simulink model "LRMate200Experimentor_ModeController"  (R2015b)
settings: Solver=FixedStepDiscrete  StartTime=0.0  StopTime=10.0  FixedStep=si.itp  RelTol=1e-3
settings Model: Creator=rluser  LastModifiedBy=Chin
settings SolverCC: EnableConcurrentExecution=on
settings DataIOCC: SaveFormat=Array
settings OptimizationCC: BlockReduction=off  OptimizeBlockIOStorage=off  BufferReuse=off  GlobalBufferReuse=off  ExpressionFolding=off  LocalBlockOutputs=off
settings DebuggingCC: SolverPrmCheckMsg=warning
settings HardwareCC: ProdBitPerPointer=32  ProdLargestAtomicFloat=None  ProdWordSize=32  ProdLongLongMode=on  ProdHWDeviceType=Generic->32-bit x86 compatible
settings RTWCC: SystemTargetFile=slrt.tlc  TemplateMakefile=slrt_default_tmf  Description=Simulink Real-Time  RTWCompilerOptimization=on
settings CodeAppCC: MaxIdLength=120
settings SimulinkRealTimeCC: GeneratePreprocessorConditionals=Disable all
settings ConfigComp: CovModelRefEnable=Off  CovSFcnEnable=off

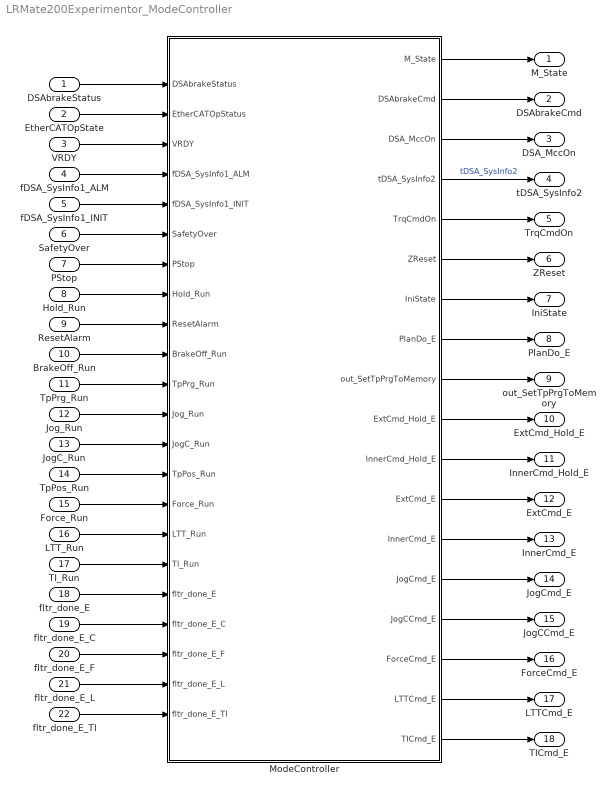
== system LRMate200Experimentor_ModeController ==
  DSAbrakeStatus : Inport
  EtherCATOpState : Inport  Port=2
  VRDY : Inport  Port=3
  fDSA_SysInfo1_ALM : Inport  Port=4
  fDSA_SysInfo1_INIT : Inport  Port=5
  SafetyOver : Inport  Port=6
  PStop : Inport  Port=7
  Hold_Run : Inport  Port=8
  ResetAlarm : Inport  Port=9
  BrakeOff_Run : Inport  Port=10
  TpPrg_Run : Inport  Port=11
  Jog_Run : Inport  Port=12
  JogC_Run : Inport  Port=13
  TpPos_Run : Inport  Port=14
  Force_Run : Inport  Port=15
  LTT_Run : Inport  Port=16
  TI_Run : Inport  Port=17
  fltr_done_E : Inport  Port=18
  fltr_done_E_C : Inport  Port=19
  fltr_done_E_F : Inport  Port=20
  fltr_done_E_L : Inport  Port=21
  fltr_done_E_TI : Inport  Port=22
  ModeController : Stateflow chart  TreatAsAtomicUnit=on
  M_State : Outport
  DSAbrakeCmd : Outport  Port=2
  DSA_MccOn : Outport  Port=3
  tDSA_SysInfo2 : Outport  Port=4
  TrqCmdOn : Outport  Port=5
  ZReset : Outport  Port=6
  IniState : Outport  Port=7
  PlanDo_E : Outport  Port=8
  out_SetTpPrgToMemory : Outport  Port=9
  ExtCmd_Hold_E : Outport  Port=10
  InnerCmd_Hold_E : Outport  Port=11
  ExtCmd_E : Outport  Port=12
  InnerCmd_E : Outport  Port=13
  JogCmd_E : Outport  Port=14
  JogCCmd_E : Outport  Port=15
  ForceCmd_E : Outport  Port=16
  LTTCmd_E : Outport  Port=17
  TICmd_E : Outport  Port=18
  wires:
  ModeController/1(M_State) -> M_State/1
  ModeController/2(DSAbrakeCmd) -> DSAbrakeCmd/1
  ModeController/3(DSA_MccOn) -> DSA_MccOn/1
  ModeController/4(tDSA_SysInfo2) -> tDSA_SysInfo2/1  "tDSA_SysInfo2"
  ModeController/5(TrqCmdOn) -> TrqCmdOn/1
  ModeController/6(ZReset) -> ZReset/1
  DSAbrakeStatus/1 -> ModeController/1(DSAbrakeStatus)
  EtherCATOpState/1 -> ModeController/2(EtherCATOpStatus)
  VRDY/1 -> ModeController/3(VRDY)
  fDSA_SysInfo1_ALM/1 -> ModeController/4(fDSA_SysInfo1_ALM)
  fDSA_SysInfo1_INIT/1 -> ModeController/5(fDSA_SysInfo1_INIT)
  SafetyOver/1 -> ModeController/6(SafetyOver)
  PStop/1 -> ModeController/7(PStop)
  Hold_Run/1 -> ModeController/8(Hold_Run)
  ResetAlarm/1 -> ModeController/9(ResetAlarm)
  BrakeOff_Run/1 -> ModeController/10(BrakeOff_Run)
  TpPrg_Run/1 -> ModeController/11(TpPrg_Run)
  Jog_Run/1 -> ModeController/12(Jog_Run)
  JogC_Run/1 -> ModeController/13(JogC_Run)
  TpPos_Run/1 -> ModeController/14(TpPos_Run)
  Force_Run/1 -> ModeController/15(Force_Run)
  LTT_Run/1 -> ModeController/16(LTT_Run)
  ModeController/7(IniState) -> IniState/1
  ModeController/8(PlanDo_E) -> PlanDo_E/1
  ModeController/9(out_SetTpPrgToMemory) -> out_SetTpPrgToMemory/1
  ModeController/10(ExtCmd_Hold_E) -> ExtCmd_Hold_E/1
  ModeController/11(InnerCmd_Hold_E) -> InnerCmd_Hold_E/1
  ModeController/12(ExtCmd_E) -> ExtCmd_E/1
  ModeController/13(InnerCmd_E) -> InnerCmd_E/1
  ModeController/14(JogCmd_E) -> JogCmd_E/1
  ModeController/15(JogCCmd_E) -> JogCCmd_E/1
  ModeController/16(ForceCmd_E) -> ForceCmd_E/1
  ModeController/17(LTTCmd_E) -> LTTCmd_E/1
  TI_Run/1 -> ModeController/17(TI_Run)
  fltr_done_E/1 -> ModeController/18(fltr_done_E)
  fltr_done_E_C/1 -> ModeController/19(fltr_done_E_C)
  fltr_done_E_F/1 -> ModeController/20(fltr_done_E_F)
  fltr_done_E_L/1 -> ModeController/21(fltr_done_E_L)
  fltr_done_E_TI/1 -> ModeController/22(fltr_done_E_TI)
  ModeController/18(TICmd_E) -> TICmd_E/1

== stateflow chart LRMate200Experimentor_ModeController/ModeController ==
  settings: updateMethod=DISCRETE  sampleTime=si.itp
  state Mode [parallel]
    settings: executionOrder=1
    state WatingForEtherCATReady
      en:M_State=-95;
      TrqCmdOn=0;
      ZReset=1;
      DSAbrakeCmd=0;
      DSA_MccOn=0;
    state INIT_DataCommArea
      en: M_State=-93;
      tDSA_SysInfo2=128;
    state Pstop_State
      state Alarm
        en:M_State=-80;
        TrqCmdOn=0;
        ZReset=1;
      state BrakeOn
        en:M_State=-82;
        DSAbrakeCmd=0;
      state MccOn
        en:M_State=-84;
        DSA_MccOn=1;
      state MccOff
        en:
        M_State=-78;
        DSA_MccOn=0;
      state ResetAlarm1
        en: M_State=-91;
        tDSA_SysInfo2=8;
      state ResetAlarm2
        en: M_State=-89;
        tDSA_SysInfo2=0;
      Alarm -> MccOff
      ResetAlarm2 -> MccOn : [fDSA_SysInfo1_ALM==0]
      ResetAlarm1 -> ResetAlarm2
      Mode.Pstop_State.BrakeOn -> Alarm : after(20,tick)
      (junction 518) -> ResetAlarm1
      MccOff -> (junction 518) : ResetAlarm_E
      MccOn -> (junction 506) : [VRDY==1]
      (junction 506) -> (junction 507)
    state in_stroke
      state Jog_Stopping
        en:JogCmd_E;
        en:M_State=22;
      state BrakeOn
        en:M_State=4;
        DSAbrakeCmd=0;
      state Jogging
        en:JogCmd_E;
        en:M_State=21;
      state JoggingC
        en:JogCCmd_E;
        en:M_State=9921;
      state JogC_Stopping
        en:JogCCmd_E;
        en:M_State=9922;
      state TrqCmdOff
        en:M_State=1;
        TrqCmdOn=0;
        ZReset=1;
      state ForceControl_Stopping
        en:ForceCmd_E;
        en:M_State=9924;
      state ForceControl
        en:ForceCmd_E;
        en:M_State=9923;
      state BrakeOff
        state TrqCmdOn
          en:
          M_State=2;
          TrqCmdOn=1;
          ZReset=0;
        state BrakeOff
          en: DSAbrakeCmd=1;
          M_State=3;
        Mode.in_stroke.BrakeOff.TrqCmdOn -> Mode.in_stroke.BrakeOff.BrakeOff : after(1,tick)
        Mode.in_stroke.BrakeOff.BrakeOff -> (junction 510) : [DSAbrakeStatus==1]
        (junction 510) -> (junction 512) : after(50,tick)
      state LeadThroughTeaching
        en:LTTCmd_E;
        en:M_State=9925;
      state Waiting
        en:M_State=1099;
      state LTT_Stopping
        en:LTTCmd_E;
        en:M_State=9926;
      state TiltInsertion
        en:TICmd_E;
        en:M_State=9927;
      state SetTpPos
        en:  out_SetTpPrgToMemory;
      state TI_Stopping1
        en:TICmd_E;
        en:M_State=9928;
      state IniPosMove_Running1
        en: PlanDo_E;
        InnerCmd_E;
        IniState = 1;
        M_State=9931;
      state SetTpPrg
        en:  out_SetTpPrgToMemory;
      state IniPosMove_Running
        en: PlanDo_E;
        InnerCmd_E;
        IniState = 0;
        M_State=31;
      state Hold_Running
        en:
        M_State=40;
      state TpPrg__Running
        en:
        M_State=33;
        ExtCmd_E;
      Jogging -> Jog_Stopping : Jog_E
      Mode.in_stroke.BrakeOn -> TrqCmdOff : after(10,tick)
      Waiting -> Jogging [order 4] : Jog_E
      Waiting -> JoggingC [order 6] : JogC_E
      Jog_Stopping -> Waiting : [hasChanged(fltr_done_E)]
      Waiting -> Mode.in_stroke.BrakeOn [order 7] : Brake_E
      JoggingC -> JogC_Stopping : JogC_E
      (default) -> (junction 426)
      (junction 426) -> TrqCmdOff
      JogC_Stopping -> Waiting : [hasChanged(fltr_done_E_C)]
      ForceControl -> ForceControl_Stopping : Force_E
      TrqCmdOff -> Mode.in_stroke.BrakeOff.TrqCmdOn : BrakeOff_E
      ForceControl_Stopping -> Waiting : [hasChanged(fltr_done_E_F)]
      Waiting -> ForceControl [order 5] : Force_E
      LeadThroughTeaching -> LTT_Stopping : LTT_E
      Waiting -> LeadThroughTeaching [order 8] : LTT_E
      LTT_Stopping -> Waiting : [hasChanged(fltr_done_E_L)]
      Waiting -> TiltInsertion [order 3] : TI_E
      (junction 188) -> Waiting
      Waiting -> (junction 186) [order 1] : TpPrg_E
      IniPosMove_Running1 -> Waiting : [hasChanged(fltr_done_E)]
      Waiting -> SetTpPos [order 2] : TpPos_E
      TI_Stopping1 -> Waiting : [hasChanged(fltr_done_E_TI)]
      TiltInsertion -> TI_Stopping1 : TI_E
      Hold_Running -> (junction 188) : [hasChanged(fltr_done_E)]
      (junction 177) -> (junction 188)
      (junction 512) -> (junction 180)
      SetTpPos -> IniPosMove_Running1
      (junction 180) -> (junction 177)
      TpPrg__Running -> (junction 177) [order 1] : [hasChanged(fltr_done_E)]
      (junction 598) -> (junction 177)
      (junction 186) -> SetTpPrg
      SetTpPrg -> IniPosMove_Running
      IniPosMove_Running -> Hold_Running [order 2] : Hold_E
          | {InnerCmd_Hold_E;}
      (junction 175) -> Hold_Running
      IniPosMove_Running -> TpPrg__Running [order 1] : [hasChanged(fltr_done_E)]
      TpPrg__Running -> (junction 175) [order 2] : Hold_E
          | {ExtCmd_Hold_E;}
    state out_stroke
      state TrqCmdOff1
        en:M_State=201;
        TrqCmdOn=0;
        ZReset=1;
      state BrakeOn1
        en:M_State=204;
        DSAbrakeCmd=0;
      state BrakeOff1
        state TrqCmdOn
          en:
          M_State=202;
          TrqCmdOn=1;
          ZReset=0;
        state BrakeOff
          en: DSAbrakeCmd=1;
          M_State=203;
        Mode.out_stroke.BrakeOff1.TrqCmdOn -> Mode.out_stroke.BrakeOff1.BrakeOff : after(1,tick)
        Mode.out_stroke.BrakeOff1.BrakeOff -> (junction 524) : [DSAbrakeStatus==1]
        (junction 524) -> (junction 525) : after(50,tick)
      state Waiting1
        en:M_State=210;
      state Jogging1
        en:JogCmd_E;
        en:M_State=221;
      state Jog_Stopping1
        en:JogCmd_E;
        en:M_State=222;
      (default) -> (junction 433)
      (junction 433) -> TrqCmdOff1
      BrakeOn1 -> TrqCmdOff1 : after(10,tick)
      Waiting1 -> BrakeOn1 [order 2] : Brake_E
      TrqCmdOff1 -> Mode.out_stroke.BrakeOff1.TrqCmdOn : BrakeOff_E
      (junction 485) -> (junction 487) [order 1] : [SafetyOver==0]
      Waiting1 -> (junction 485) [order 3] : ResetAlarm_E
      (junction 485) -> Waiting1 [order 2]
      (junction 487) -> (junction 501)
      Waiting1 -> Jogging1 [order 1] : Jog_E
      (junction 461) -> Waiting1
      Jog_Stopping1 -> Waiting1 : [hasChanged(fltr_done_E)]
      Jogging1 -> Jog_Stopping1 : Jog_E
      (junction 525) -> (junction 460)
      (junction 460) -> (junction 461)
      (junction 501) -> (junction 504)
    (default) -> WatingForEtherCATReady
    WatingForEtherCATReady -> INIT_DataCommArea : [EtherCATOpStatus==8]
    INIT_DataCommArea -> (junction 518) : [fDSA_SysInfo1_INIT==1]
    (junction 406) -> Mode.Pstop_State.BrakeOn
    (junction 401) -> (junction 406)
    (junction 507) -> (junction 417)
    (junction 417) -> (junction 423) [order 2]
    (junction 417) -> (junction 419) [order 1] : [SafetyOver==0]
    (junction 423) -> out_stroke : % [SafetyOver==1]
    (junction 419) -> in_stroke
    in_stroke -> (junction 401) [order 1] : PStop_E
    out_stroke -> (junction 401) [order 1] : PStop_E
    (junction 403) -> (junction 401)
    in_stroke -> (junction 403) [order 2] : [fDSA_SysInfo1_ALM==1]
    (junction 439) -> (junction 403)
    in_stroke -> (junction 439) [order 3] : [SafetyOver~=0]
    (junction 594) -> (junction 439)
    in_stroke -> (junction 594) [order 4] : [VRDY==0]
        | %Press TP P-STOP Button
    out_stroke -> (junction 594) [order 2] : [VRDY==0]
    (junction 504) -> (junction 598)
  state Buttons [group]
    state Button_BreakOff [parallel]
      settings: executionOrder=1
      state S0
      Buttons.Button_BreakOff.S0 -> Buttons.Button_BreakOff.S0 : [hasChangedTo(BrakeOff_Run,1)]
          | {send(BrakeOff_E,Mode);}
      (default) -> Buttons.Button_BreakOff.S0
    state Button_ResetAlarm [parallel]
      settings: executionOrder=6
      state S0
      Buttons.Button_ResetAlarm.S0 -> Buttons.Button_ResetAlarm.S0 : [hasChanged(ResetAlarm)]
          | {send(ResetAlarm_E,Mode);}
      (default) -> Buttons.Button_ResetAlarm.S0
    state Button_LeadThroughTeaching [parallel]
      settings: executionOrder=11
      state S0
      Buttons.Button_LeadThroughTeaching.S0 -> Buttons.Button_LeadThroughTeaching.S0 : [hasChanged(LTT_Run)]
          | {send(LTT_E,Mode);}
      (default) -> Buttons.Button_LeadThroughTeaching.S0
    state Button_Jog [parallel]
      settings: executionOrder=2
      state S0
      Buttons.Button_Jog.S0 -> Buttons.Button_Jog.S0 : [hasChanged(Jog_Run)]
          | {send(Jog_E,Mode);}
      (default) -> Buttons.Button_Jog.S0
    state Button_PStop [parallel]
      settings: executionOrder=7
      state S0
      Buttons.Button_PStop.S0 -> Buttons.Button_PStop.S0 : [hasChanged(PStop)]
          | {send(PStop_E,Mode);}
      (default) -> Buttons.Button_PStop.S0
    state Button_TiltInsertion [parallel]
      settings: executionOrder=12
      state S0
      Buttons.Button_TiltInsertion.S0 -> Buttons.Button_TiltInsertion.S0 : [hasChanged(TI_Run)]
          | {send(TI_E,Mode);}
      (default) -> Buttons.Button_TiltInsertion.S0
    state Button_TpPrg [parallel]
      settings: executionOrder=3
      state S0
      Buttons.Button_TpPrg.S0 -> Buttons.Button_TpPrg.S0 : [hasChangedTo(TpPrg_Run,1)]
          | {send(TpPrg_E,Mode);}
      (default) -> Buttons.Button_TpPrg.S0
    state Button_JogC [parallel]
      settings: executionOrder=8
      state S0
      Buttons.Button_JogC.S0 -> Buttons.Button_JogC.S0 : [hasChanged(JogC_Run)]
          | {send(JogC_E,Mode);}
      (default) -> Buttons.Button_JogC.S0
    state Button_Hold [parallel]
      settings: executionOrder=4
      state S0
      Buttons.Button_Hold.S0 -> Buttons.Button_Hold.S0 : [hasChanged(Hold_Run)]
          | {send(Hold_E,Mode);}
      (default) -> Buttons.Button_Hold.S0
    state Button_TpPos [parallel]
      settings: executionOrder=9
      state S0
      Buttons.Button_TpPos.S0 -> Buttons.Button_TpPos.S0 : [hasChangedTo(TpPos_Run,1)]
          | {send(TpPos_E,Mode);}
      (default) -> Buttons.Button_TpPos.S0
    state Button_BrakeOn [parallel]
      settings: executionOrder=5
      state S0
      Buttons.Button_BrakeOn.S0 -> Buttons.Button_BrakeOn.S0 : [hasChangedTo(BrakeOff_Run,0)]
          | {send(Brake_E,Mode);}
      (default) -> Buttons.Button_BrakeOn.S0
    state Button_ForceControl [parallel]
      settings: executionOrder=10
      state S0
      Buttons.Button_ForceControl.S0 -> Buttons.Button_ForceControl.S0 : [hasChanged(Force_Run)]
          | {send(Force_E,Mode);}
      (default) -> Buttons.Button_ForceControl.S0
  data: DSAbrakeStatus input double size=1; EtherCATOpStatus input double size=1; VRDY input boolean size=1 =0; fDSA_SysInfo1_ALM input boolean; fDSA_SysInfo1_INIT input boolean; SafetyOver input double size=1; PStop input double; Hold_Run input double; ResetAlarm input double; BrakeOff_Run input double; TpPrg_Run input double; Jog_Run input double; JogC_Run input double; TpPos_Run input double; Force_Run input double; LTT_Run input double; TI_Run input double; M_State output double size=1 =0; fltr_done_E input boolean; DSAbrakeCmd output double size=1 =0; DSA_MccOn output double size=1 =0; tDSA_SysInfo2 output double size=1 =0; TrqCmdOn output boolean size=1 =0; ZReset output boolean size=1 =0; fltr_done_E_C input boolean; IniState output double; fltr_done_E_F input boolean; fltr_done_E_L input boolean; fltr_done_E_TI input boolean
  events: BrakeOff_E local EITHER_EDGE_EVENT; TpPrg_E local EITHER_EDGE_EVENT; Hold_E local FUNCTION_CALL_EVENT; PlanDo_E output EITHER_EDGE_EVENT; out_SetTpPrgToMemory output EITHER_EDGE_EVENT; ExtCmd_Hold_E output EITHER_EDGE_EVENT; InnerCmd_Hold_E output EITHER_EDGE_EVENT; ExtCmd_E output EITHER_EDGE_EVENT; InnerCmd_E output EITHER_EDGE_EVENT; Jog_E local FUNCTION_CALL_EVENT; JogCmd_E output EITHER_EDGE_EVENT; Brake_E local FUNCTION_CALL_EVENT; ResetAlarm_E local FUNCTION_CALL_EVENT; PStop_E local FUNCTION_CALL_EVENT; JogC_E local FUNCTION_CALL_EVENT; JogCCmd_E output EITHER_EDGE_EVENT; TpPos_E local FUNCTION_CALL_EVENT; ForceCmd_E output EITHER_EDGE_EVENT; Force_E local FUNCTION_CALL_EVENT; LTTCmd_E output EITHER_EDGE_EVENT; LTT_E local FUNCTION_CALL_EVENT; TICmd_E output EITHER_EDGE_EVENT; TI_E local FUNCTION_CALL_EVENT
